simulink model "OFDMwithQPSK"  (R2021a)
settings: Solver=VariableStepAuto  StartTime=0.0  StopTime=10.0  RelTol=1e-3
libraries: commdigbbndpm3 x2, commofdm x2, commchan3 x1, commrandsrc3 x1, commsink2 x1, impairlib x1
settings Model: Creator=Ian  LastModifiedBy=Ian

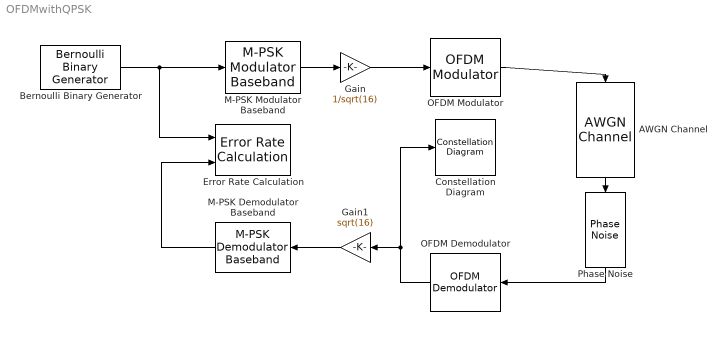
== system OFDMwithQPSK ==
  AWGN Channel : commchan3/AWGN Channel  InputProcessing=Columns as channels (frame based)  seed=42  noiseMode="Signal to noise ratio  (Eb/No)"  EbNodB=EbNo  EsNodB=10  SNRdB=10  bitsPerSym=192  Ps=1  Tsym=64  variance=1
  Bernoulli Binary Generator : commrandsrc3/Bernoulli Binary Generator  ProbabilityOfZero=0.5  SeedSource=Parameter  Seed=42  SampleTime=1/(192*1e-3)  SamplesPerFrame=192  OutputDataType=double  SimulateUsing=Interpreted execution
  Constellation Diagram : ConstellationDiagram
  Error Rate Calculation : commsink2/Error Rate Calculation  N=0  st_delay=0  cp_mode=Entire frame  subframe=[]  PMode=Workspace  WsName=simout  RsMode2=off  stop=off  numErr=100  maxBits=1e6
  Gain : Gain  Gain=1/sqrt(16)
  Gain1 : Gain  Gain=sqrt(16)
  M-PSK Demodulator Baseband : commdigbbndpm3/M-PSK Demodulator Baseband  M=4  OutType=Bit  DecType=Hard decision  VarSource=Dialog  Variance=1  Dec=Gray  Mapping=[0:7]  Ph=pi/8  outDtype1=Inherit via internal rule  outDtype2=Inherit via internal rule  derotateFactorWordLen=16  derotateFactorDataTypeStr=Inherit: Same word length as input  derotateFactorLastDataTypeStr=Inherit: Same word length as input
  M-PSK Modulator Baseband : commdigbbndpm3/M-PSK Modulator Baseband  M=4  InType=Bit  Enc=Gray  Mapping=[0:7]  Ph=pi/8  outDtype=double  outWordLen=16  outUDDataType=sfix(16)  outFracLenMode=Best precision  outFracLen=15  outDataTypeStr=double  outLastDataTypeStr=double
  OFDM Demodulator : commofdm/OFDM Demodulator  StatePerturbationForJacobian=1.0e-05  FFTLength=128  NumGuardBandCarriers=[16; 16]  RemoveDCCarrier=off  PilotOutputPort=off  PilotCarrierIndices=[12; 26; 40; 54]  CyclicPrefixLength=16  NumSymbols=1  NumReceiveAntennas=1  SimulateUsing=Interpreted execution
      settings: SourceProductBaseCode=CM
  OFDM Modulator : commofdm/OFDM Modulator  StatePerturbationForJacobian=1.0e-05  FFTLength=128  NumGuardBandCarriers=[16; 16]  InsertDCNull=off  PilotInputPort=off  PilotCarrierIndices=[12; 26; 40; 54]  CyclicPrefixLength=16  Windowing=off  WindowLength=1  NumSymbols=1  NumTransmitAntennas=1  SimulateUsing=Interpreted execution
      settings: SourceProductBaseCode=CM
  Phase Noise : impairlib/Phase Noise  Level=[-80 -100]  FrequencyOffset=[0.01 0.02]  SampleRate=0.144  RandomStream=mt19937ar with seed  Seed=2137  SimulateUsing=Interpreted execution
      settings: SourceProductBaseCode=CM,AM,SX
  wires:
  Bernoulli Binary Generator/1 -> Error Rate Calculation/1, M-PSK Modulator Baseband/1
  M-PSK Modulator Baseband/1 -> Gain/1
  AWGN Channel/1 -> Phase Noise/1
  Gain/1 -> OFDM Modulator/1
  OFDM Modulator/1 -> AWGN Channel/1
  Phase Noise/1 -> OFDM Demodulator/1
  OFDM Demodulator/1 -> Constellation Diagram/1, Gain1/1
  Gain1/1 -> M-PSK Demodulator Baseband/1
  M-PSK Demodulator Baseband/1 -> Error Rate Calculation/2
